simulink model "Single_Phase_Transformer"  (R2019b)
settings: Solver=VariableStepAuto  StartTime=0.0  StopTime=0.05  MaxStep=0.001  RelTol=1e-3  AbsTol=1e-3  EnableMultiTasking=on
libraries: fl_lib x6, nesl_utility x3, ee_lib x1
CloseFcn:
  | try,close(h1_ssc_bridge_rectifier),end
  | clear h1_ssc_bridge_rectifier
  | 
  | 
  | clear simlog_ssc_bridge_rectifier
Description:
  | Full-Wave Bridge Rectifier
settings Model: Creator=MathWorks  LastModifiedBy=ANTO
settings SolverCC: AutoScaleAbsTol=off
settings DataIOCC: LimitDataPoints=on  SaveFormat=Array  ReturnWorkspaceOutputs=off
settings OptimizationCC: LifeSpan=inf
settings DebuggingCC: SolverPrmCheckMsg=warning  AllowSymbolicDim=off  PregeneratedLibrarySubsystemCodeDiagnostic=none  SFUnexpectedBacktrackingDiag=warning  SFNoUnconditionalDefaultTransitionDiag=warning  SFExecutionAtInitializationDiag=none  ArithmeticOperatorsInVariantConditions=warning
settings HardwareCC: ProdBitPerPointer=32  ProdBitPerSizeT=32  ProdBitPerPtrDiffT=32  ProdLargestAtomicFloat=None  ProdIntDivRoundTo=Undefined  ProdEndianess=Unspecified  ProdWordSize=32  ProdHWDeviceType=32-bit Generic
settings ModelReferenceCC: PropagateSignalLabelsOutOfModel=off
settings SFSimCC: SimUseLocalCustomCode=off  CustomCodeUndefinedFunction=UseInterfaceOnly
settings RTWCC: RTWUseLocalCustomCode=off
settings CodeAppCC: StateflowObjectComments=on
settings GRTTargetCC: TargetLangStandard=C89/C90 (ANSI)  GeneratePreprocessorConditionals=Disable all
settings ConfigComp: CovMetricSettings=dw  CovHtmlReporting=on  CovSaveCumulativeToWorkspaceVar=on  CovSaveSingleToWorkspaceVar=on  CovExternalEMLEnable=off  CovSFcnEnable=off
settings SimscapeCC: SimscapeLogType=all  SimscapeLogSimulationStatistics=on  SimscapeLogName=simlog_ssc_bridge_rectifier  SimscapeLogDataHistory=10000

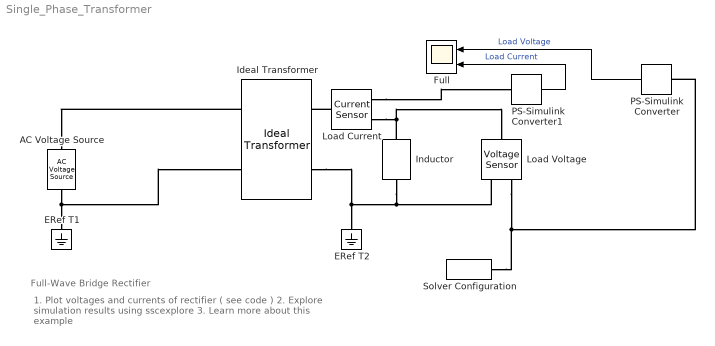
== system Single_Phase_Transformer ==
  note: 1. Plot voltages and currents of rectifier ( see code )
      | 2. Explore simulation results using sscexplore
      | 3. Learn more about this example
  note: Full-Wave Bridge Rectifier
  AC Voltage Source : fl_lib/Electrical/Electrical Sources/AC Voltage Source  amp=sqrt(2)*230 V  shift=0 deg  frequency=50 Hz  omega=0 rad/s
  ERef T1 : fl_lib/Electrical/Electrical Elements/Electrical Reference
  ERef T2 : fl_lib/Electrical/Electrical Elements/Electrical Reference
  Full : Scope  NumInputPorts=2
  Ideal Transformer : fl_lib/Electrical/Electrical Elements/Ideal Transformer  n=9.58  i1_specify=off  i1_priority=High  i1=0 A  i1_nominal_specify=off  i1_nominal_unit=A  i1_nominal_value=1  v1_specify=off  v1_priority=High  v1=0 V  v1_nominal_specify=off  v1_nominal_unit=V  v1_nominal_value=1  i2_specify=off  i2_priority=High  i2=0 A  i2_nominal_specify=off  i2_nominal_unit=A  i2_nominal_value=1  v2_specify=off  v2_priority=High  v2=0 V  v2_nominal_specify=off  v2_nominal_unit=V  v2_nominal_value=1
      settings: SourceProductName=Simscape  SourceProductBaseCode=SS
  Inductor : ee_lib/Passive/Inductor  l=0.01177 H  L_tol=20  enable_L_tol=0  tol_distribution=1  nSigma=4  r=0 Ohm  g=0 1/Ohm  enable_operating_limits=0  operating_limit_action=2  max_working_current=1 A  power_rating=1 W  enable_faults=0  fault_action=1  lambdaPercent=50  k_faulted=0.9999  turnsShort=0  openCct=0  groundShort=0  groundShortG=0 1/Ohm  tau_fault=1e-3 s  enable_temporal_fault=0  t_fault=1 s  enable_behavioral_fault=0  max_permissible_voltage=100 V  n_fail_on_voltage=1  max_permissible_current=1 A  t_fail_on_current=1 s  i_L_specify=off  i_L_priority=High  i_L=5 A  i_L_nominal_specify=off  i_L_nominal_unit=A  i_L_nominal_value=1
      settings: SourceProductName=Simscape Electrical
  Load Current : fl_lib/Electrical/Electrical Sensors/Current Sensor
  Load Voltage : fl_lib/Electrical/Electrical Sensors/Voltage Sensor
  PS-Simulink Converter : nesl_utility/PS-Simulink Converter  PhysicalDomain=network_engine_domain  SubClassName=ps_output  LeftPortType=input  RightPortType=output  PseudoPeriodic=off  Frequencies=[]  Unit=1  AffineConversion=off
  PS-Simulink Converter1 : nesl_utility/PS-Simulink Converter  PhysicalDomain=network_engine_domain  SubClassName=ps_output  LeftPortType=input  RightPortType=output  PseudoPeriodic=off  Frequencies=[]  Unit=1  AffineConversion=off
  Solver Configuration : nesl_utility/Solver Configuration  PhysicalDomain=network_engine_domain  SubClassName=solver  LeftPortType=input  RightPortType=generic  Tones=[]  Harmonics=[]  SimulateNoise=off  Profile=off  UseLocalSampling=off  EnableSwitchedLinearOptims=on  FrequencyDomain=off  UseCCode=off  RelTol=0.001  AbsTol=1e-06  MinStep=1e-09  ToWorkspace=off  RevertToSquareIcSolve=off  NumHomotopyIterations=100  PhasorMode=off  PhasorModeNumHarmonics=1  DoDC=off  ResidualTolerance=1e-9  UseLocalSolver=off  LocalSolverChoice=NE_BACKWARD_EULER_ADVANCER  LocalSolverSampleTime=.001  DoFixedCost=off  MaxNonlinIter=3  MaxModeIter=2  LinearAlgebra=auto  EquationFormulation=NE_TIME_EF  DelaysMemoryBudget=1024  AutomaticFiltering=on  FilteringTimeConstant=0.001  PartitionStorageMethod=AS_NEEDED  PartitionMemoryBudget=1024  PartitionMethod=FAST
  wires:
  PS-Simulink Converter/1 -> Full/1  "Load Voltage"
  PS-Simulink Converter1/1 -> Full/2  "Load Current"
  connections:
  AC Voltage Source/RConn1 -- ERef T1/LConn1 -- Ideal Transformer/LConn2
  Ideal Transformer/RConn2 -- Load Voltage/RConn2 -- Inductor/RConn1 -- ERef T2/LConn1
  Load Voltage/RConn1 -- Solver Configuration/RConn1 -- PS-Simulink Converter/LConn1
  Ideal Transformer/LConn1 -- AC Voltage Source/LConn1
  Inductor/LConn1 -- Load Voltage/LConn1 -- Load Current/RConn2
  Load Current/LConn1 -- Ideal Transformer/RConn1
  Load Current/RConn1 -- PS-Simulink Converter1/LConn1
